simulink model "ARDrone2_ContinuousSimulation"  (R2014b)
settings: Solver=ode45  StartTime=0.0  StopTime=10.0  RelTol=1e-3
settings Model: Creator=m  LastModifiedBy=m
settings DebuggingCC: UnderspecifiedInitializationDetection=Classic  MergeDetectMultiDrivingBlocksExec=none  StateNameClashWarn=warning

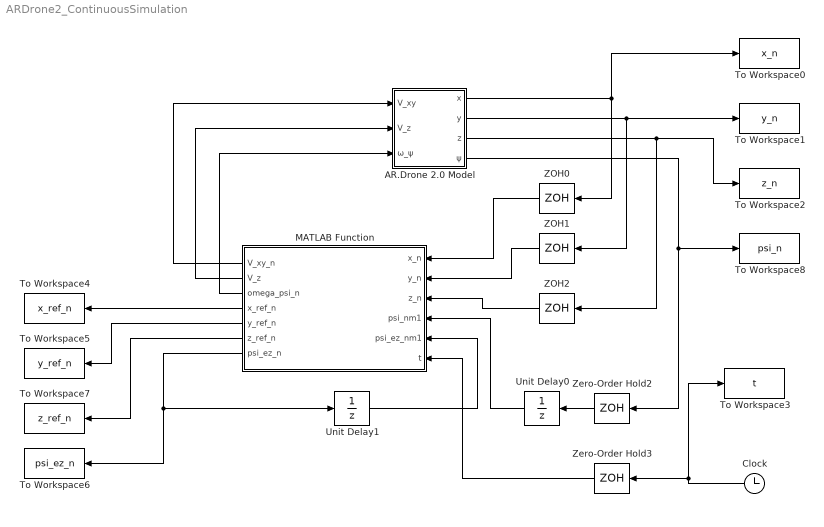
== system ARDrone2_ContinuousSimulation ==
  AR.Drone 2.0 Model : Subsystem
  Clock : Clock
  MATLAB Function : MATLAB Function  TreatAsAtomicUnit=on
  To Workspace0 : ToWorkspace  VariableName=x_n  SampleTime=0.1
  To Workspace1 : ToWorkspace  VariableName=y_n  SampleTime=0.1
  To Workspace2 : ToWorkspace  VariableName=z_n  SampleTime=0.1
  To Workspace3 : ToWorkspace  VariableName=t  SampleTime=0.1
  To Workspace4 : ToWorkspace  VariableName=x_ref_n  SampleTime=0.1
  To Workspace5 : ToWorkspace  VariableName=y_ref_n  SampleTime=0.1
  To Workspace6 : ToWorkspace  VariableName=psi_ez_n  SampleTime=0.1
  To Workspace7 : ToWorkspace  VariableName=z_ref_n  SampleTime=0.1
  To Workspace8 : ToWorkspace  VariableName=psi_n  SampleTime=0.1
  Unit Delay0 : UnitDelay  SampleTime=-1
  Unit Delay1 : UnitDelay  SampleTime=-1
  ZOH0 : ZeroOrderHold  SampleTime=0.1
  ZOH1 : ZeroOrderHold  SampleTime=0.1
  ZOH2 : ZeroOrderHold  SampleTime=0.1
  Zero-Order Hold2 : ZeroOrderHold  SampleTime=0.1
  Zero-Order Hold3 : ZeroOrderHold  SampleTime=0.1
  wires:
  AR.Drone 2.0 Model/2(y) -> To Workspace1/1, ZOH1/1
  AR.Drone 2.0 Model/4(ψ) -> Zero-Order Hold2/1, To Workspace8/1
  Clock/1 -> Zero-Order Hold3/1, To Workspace3/1
  AR.Drone 2.0 Model/1(x) -> To Workspace0/1, ZOH0/1
  ZOH0/1 -> MATLAB Function/1(x_n)
  ZOH1/1 -> MATLAB Function/2(y_n)
  Zero-Order Hold2/1 -> Unit Delay0/1
  Unit Delay0/1 -> MATLAB Function/4(psi_nm1)
  Zero-Order Hold3/1 -> MATLAB Function/6(t)
  Unit Delay1/1 -> MATLAB Function/5(psi_ez_nm1)
  MATLAB Function/1(V_xy_n) -> AR.Drone 2.0 Model/1(V_xy)
  MATLAB Function/3(omega_psi_n) -> AR.Drone 2.0 Model/3(ω_ψ)
  MATLAB Function/4(x_ref_n) -> To Workspace4/1
  MATLAB Function/5(y_ref_n) -> To Workspace5/1
  AR.Drone 2.0 Model/3(z) -> ZOH2/1, To Workspace2/1
  ZOH2/1 -> MATLAB Function/3(z_n)
  MATLAB Function/6(z_ref_n) -> To Workspace7/1
  MATLAB Function/7(psi_ez_n) -> Unit Delay1/1, To Workspace6/1
  MATLAB Function/2(V_z) -> AR.Drone 2.0 Model/2(V_z)

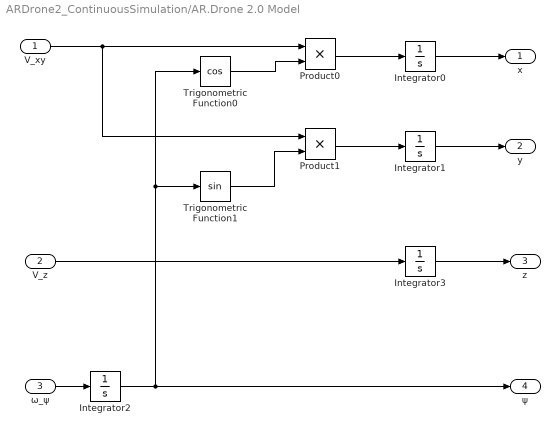
== system ARDrone2_ContinuousSimulation/AR.Drone 2.0 Model ==
  V_xy : Inport
  V_z : Inport  Port=2
  ω_ψ : Inport  Port=3
  Integrator0 : Integrator
  Integrator1 : Integrator
  Integrator2 : Integrator  InitialCondition=0.01
  Integrator3 : Integrator
  Product0 : Product
  Product1 : Product
  Trigonometric Function0 : Trigonometry  Operator=cos
  Trigonometric Function1 : Trigonometry
  x : Outport
  y : Outport  Port=2
  z : Outport  Port=3
  ψ : Outport  Port=4
  wires:
  Integrator2/1 -> ψ/1, Trigonometric Function0/1, Trigonometric Function1/1
  Product0/1 -> Integrator0/1
  ω_ψ/1 -> Integrator2/1
  V_xy/1 -> Product1/1, Product0/1
  Product1/1 -> Integrator1/1
  Trigonometric Function0/1 -> Product0/2
  Trigonometric Function1/1 -> Product1/2
  Integrator1/1 -> y/1
  Integrator0/1 -> x/1
  Integrator3/1 -> z/1
  V_z/1 -> Integrator3/1

== matlab function ARDrone2_ContinuousSimulation/MATLAB Function ==
  data: V_xy_n output; V_z output; omega_psi_n output; x_ref_n output; y_ref_n output; z_ref_n output; x_n input; y_n input; z_n input; psi_nm1 input; psi_ez_nm1 input; t input; psi_ez_n output
%%%%%%%%%%%%%%%%%%%%%%%%%% AR.DRONE 2.0 CONTROLLER %%%%%%%%%%%%%%%%%%%%%%%%
%%%%%%%%%%%%%%%%%%%%%%%%%%%%%%%%%%%%%%%%%%%%%%%%%%%%%%%%%%%%%%%%%%%%%%%%%%%
function [V_xy_n, V_z, omega_psi_n, x_ref_n, y_ref_n, z_ref_n, psi_ez_n]= ...
    controller(x_n, y_n, z_n, psi_nm1, psi_ez_nm1, t)
%% Constants
% Sample Time 
T0 = 0.1;
% Controller Constants:
% these constants take values between 0 and 1 (non-inclusive)
K_V_XY = 0.91;
K_V_Z = 0.91;
K_OMEGA_PSI = 0.91;
% others
V_REF = 0.200;
PSI_REF = pi/4;
Z = 1.2;

%% Controller Logic
% The reference trajectory is the preestablish trajectory
% the quadrotor is supposed to follow.

% Reference Trajectory at n
x_ref_n = 0.1 + V_REF * cos(PSI_REF) * t;
y_ref_n = 0.1 + V_REF * sin(PSI_REF) * t * t;
z_ref_n = Z;
% Reference Trajectory at n + 1
x_ref_np1 = 0.1 + V_REF * cos(PSI_REF) * (t + T0);
y_ref_np1 = 0.1 + V_REF * sin(PSI_REF) * (t + T0) ^ 2;
z_ref_np1 = Z;

psi_ez_n = atan((y_ref_np1 - K_V_XY * (y_ref_n - y_n) - y_n) /...
    (x_ref_np1 - K_V_XY * (x_ref_n - x_n) - x_n));

% Control Actions
V_xy_n = (1 / T0) * ((x_ref_np1 - K_V_XY * (x_ref_n - x_n) - x_n) ...
    * cos(psi_ez_n) + (y_ref_np1 - K_V_XY * (y_ref_n - y_n) - y_n)...
    * sin(psi_ez_n));

V_z = (1 / T0) * (z_ref_np1 - K_V_Z * (z_ref_n - z_n) - z_n);

omega_psi_n = (1 / T0) * (psi_ez_n - K_OMEGA_PSI * (psi_ez_nm1 ...
    - psi_nm1) - psi_nm1);
%%%%%%%%%%%%%%%%%%%%%%%%%%%%%%%%%%%%%%%%%%%%%%%%%%%%%%%%%%%%%%%%%%%%%%%%%%%
